simulink model "AA1111"  (R2018b)
settings: Solver=ode3  StartTime=0.0  StopTime=6000  FixedStep=T  RelTol=1e-3
PreLoadFcn:
  | Initial_LZ04
InitFcn:
  | Initial_LZ04
values from neighbouring files (symbols this model uses):
  Abg_GyroA = [0 0 1;0 1 0;-1 0 0]    [Initial_LZ04.m]
  Abg_GyroB = angle2dcm(-pi*3/4,0,-58/180*pi,'ZYX')    [Initial_LZ04.m]
  Abm_MmA = [0 -1 0;1 0 0;0 0 1]    [Initial_LZ04.m]
  Abm_MmB = [0 -1 0;1 0 0;0 0 1]    [Initial_LZ04.m]
  Att0 = 1*[80 0 0]'*pi/180    [Initial_LZ04.m]
  FixErr_StA = [15;15;15]*0*Kg_FixErr_St    [Initial_LZ04.m]
  FixErr_StB = ([15;15;15]*0+[10800;0;0])*Kg_FixErr_St    [Initial_LZ04.m]
  Fw_Mode = FW_Block(8,1)    [Initial.m]    (also in Initial_LZ04.m = 2)
  Fw_tao = 0.3    [Initial_LZ04.m]
  FwHmax = 4    [Initial_LZ04.m]
  FwTmax = FwTmax0    (= 0.05)    [Initial_LZ04.m]
  H0 = 0*[2;-2;-2;0]    [Initial_LZ04.m]
  Ib0_0 = [117.6 -1.39e-1 -1.14;-1.39e-1 101.9 -8.37e-2;-1.14 -8.37e-2 109.0]    [Initial_LZ04.m]
  jw = 0.0064    [Initial_LZ04.m]
  Matrix_I0 = [sin(50/180*pi)*cos(45/180*pi) -sin(50/180*pi)*cos(45/180*pi) -sin(50/180*pi)*cos(45/180*pi) sin(50/180*pi)*cos(45/180*pi);           sin(50/180*pi)*sin(45/180*pi) sin(50/180*pi)*sin(45/180*pi) -sin(50/180*pi)*sin(45/180*pi) -sin(50/180*pi)*sin(45/180*pi);           cos(50/180*pi) cos(50/180*pi) cos(50/180*pi) cos(50/180*pi)]    [Initial_LZ04.m]
  MtInfluence = 0    [Initial_LZ04.m]
  mu = 3.9860044e14    (= 398600440000000)    [Initial_LZ04.m]    (also in ZZ_User_Att.m)
  Ngc1 = [0.01;-0.02;-0.03]*Kg_Drift_Gyro*1+0*[0.001;-0.001;-0.001]    [Initial_LZ04.m]
  Ngc2 = [-0.02;0.01;-0.03]*Kg_Drift_Gyro    [Initial_LZ04.m]
  NgwxA = 0.005/60*sqrt(1/T_ctrl)*3*Kg_Noise_Gyro    [Initial_LZ04.m]
  NgwxB = 0.02/60*sqrt(1/T_ctrl)*3*Kg_Noise_Gyro    [Initial_LZ04.m]
  Noise_Mm = 7e-5*Kg_Noise_Mm    (= 7e-05)    [Initial_LZ04.m]
  Noise_StA = [3;3;30]*Kg_Noise_St    [Initial_LZ04.m]
  Noise_StB = [3;3;30]*Kg_Noise_St    [Initial_LZ04.m]
  OpenLoop_Att = 0    [Initial_LZ04.m]
  OpenLoop_Obt = 0    [Initial_LZ04.m]
  Qbs_StAFix = quatmultiply(angle2quat(pi,0,0,'XYZ'),angle2quat(-40/180*pi,20/180*pi,0,'XYZ'))    [Initial_LZ04.m]
  Qbs_StBFix = quatmultiply(angle2quat(pi,0,0,'XYZ'),angle2quat(40/180*pi,20/180*pi,0,'XYZ'))    [Initial_LZ04.m]
  Re = 6371.14e+3    (= 6371140)    [Initial.m]    (also in Initial_LZ04.m; ZZ_SystemApp.m)
  StartTime = [Year Month Day Hour Min Sec]'    [Initial_LZ04.m]
  T = T_PID - MainI.*[a_f/180*pi;0;0]    [Att_Ctrl.m]    (also in Initial_LZ04.m = 0.125; ZZ_Att.m = Tc(Axis))
  T_ctrl = 0.25    [Initial_LZ04.m]
  vx0 = sqrt(mu/a/(1-e^2))*(-sin(f)*sp(1)+(e+cos(f))*sq(1))    [Initial_LZ04.m]
  vy0 = sqrt(mu/a/(1-e^2))*(-sin(f)*sp(2)+(e+cos(f))*sq(2))    [Initial_LZ04.m]
  vz0 = sqrt(mu/a/(1-e^2))*(-sin(f)*sp(3)+(e+cos(f))*sq(3))    [Initial_LZ04.m]
  W_bi0 = 1*[0;-w0;0]+0*[2;-2;2]*pi/180    [Initial_LZ04.m]
  x0 = r0*(cos(omg+f)*cos(OMG)-sin(omg+f)*cos(i)*sin(OMG))    [Initial_LZ04.m]
  y0 = r0*(cos(omg+f)*sin(OMG)+sin(omg+f)*cos(i)*cos(OMG))    [Initial_LZ04.m]
  z0 = r0*sin(omg+f)*sin(i)    [Initial_LZ04.m]
undefined symbols (not defined in the file or in its folder): DiscIntNeverNeededParam, omegawXa
libraries: sharedutil x26, aerolibutil x15, simulink x12, sharedtransform x9, dspinverses x3, aerolibobsolete x1, vrlib x1
(part 2 of 3)

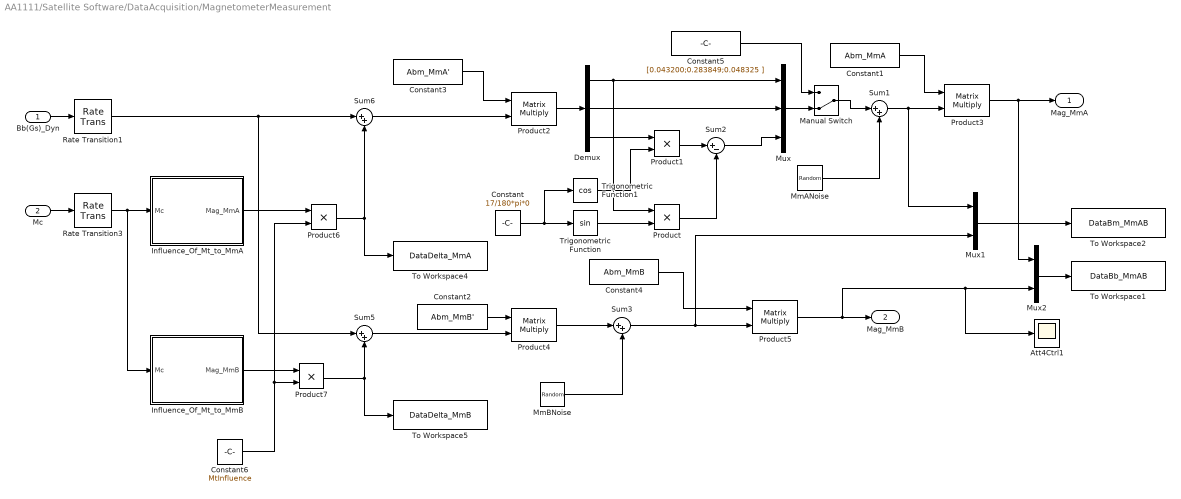
== system AA1111/Satellite Software/DataAcquisition/MagnetometerMeasurement ==
  Bb(Gs)_Dyn : Inport
  Mc : Inport  Port=2
  Att4Ctrl1 : Scope
  Constant : Constant  Value=17/180*pi*0
  Constant1 : Constant  Value=Abm_MmA
  Constant2 : Constant  Value=Abm_MmB'
  Constant3 : Constant  Value=Abm_MmA'
  Constant4 : Constant  Value=Abm_MmB
  Constant5 : Constant  Value=|
      | [0.043200;0.283849;0.048325
      | ]
  Constant6 : Constant  Value=MtInfluence
  Demux : Demux  Outputs=3
  Influence_Of_Mt_to_MmA : Subsystem
  Influence_Of_Mt_to_MmB : Subsystem
  Manual Switch : ManualSwitch  CurrentSetting=0
  MmANoise : RandomNumber  Mean=[0;0;0]  Variance=[(Noise_Mm/3)^2;(Noise_Mm/3)^2;(Noise_Mm/3)^2]  Seed=[100;111;112]  SampleTime=T_ctrl
  MmBNoise : RandomNumber  Mean=[0;0;0]  Variance=[(Noise_Mm/3)^2;(Noise_Mm/3)^2;(Noise_Mm/3)^2]  Seed=[10;11;12]  SampleTime=T_ctrl
  Mux : Mux  Inputs=3
  Mux1 : Mux  Inputs=2
  Mux2 : Mux  Inputs=2
  Product{,1,6..7} (4 alike) : Product  RndMeth=Zero
  Product{2..5} (4 alike) : Product  Multiplication=Matrix(*)  RndMeth=Zero
  Rate Transition1 : RateTransition  OutPortSampleTime=T_ctrl
  Rate Transition3 : RateTransition  OutPortSampleTime=T_ctrl
  Sum{1,3,5..6} (4 alike) : Sum  Inputs=|++
  Sum2 : Sum  Inputs=|+-
  To Workspace1 : ToWorkspace  VariableName=DataBb_MmAB  SampleTime=T_ctrl
  To Workspace2 : ToWorkspace  VariableName=DataBm_MmAB  SampleTime=T_ctrl
  To Workspace4 : ToWorkspace  VariableName=DataDelta_MmA  SampleTime=T_ctrl
  To Workspace5 : ToWorkspace  VariableName=DataDelta_MmB  SampleTime=T_ctrl
  Trigonometric Function : Trigonometry
  Trigonometric Function1 : Trigonometry  Operator=cos
  Mag_MmA : Outport
  Mag_MmB : Outport  Port=2
  wires:
  Demux/1 -> Mux/1, Product/1
  Demux/2 -> Mux/2
  Constant/1 -> Trigonometric Function/1, Trigonometric Function1/1
  Trigonometric Function/1 -> Product/2
  Demux/3 -> Product1/1
  Trigonometric Function1/1 -> Product1/2
  Product1/1 -> Sum2/1
  Product/1 -> Sum2/2
  Sum2/1 -> Mux/3
  Constant3/1 -> Product2/1
  Product2/1 -> Demux/1
  Bb(Gs)_Dyn/1 -> Rate Transition1/1
  Sum1/1 -> Product3/2, Mux1/1
  MmANoise/1 -> Sum1/2
  Constant2/1 -> Product4/1
  MmBNoise/1 -> Sum3/2
  Product4/1 -> Sum3/1
  Constant4/1 -> Product5/1
  Sum3/1 -> Product5/2, Mux1/2
  Product5/1 -> Mag_MmB/1, Mux2/2, Att4Ctrl1/1
  Constant1/1 -> Product3/1
  Product3/1 -> Mag_MmA/1, Mux2/1
  Mux1/1 -> To Workspace2/1
  Mux2/1 -> To Workspace1/1
  Mux/1 -> Manual Switch/2
  Manual Switch/1 -> Sum1/1
  Constant5/1 -> Manual Switch/1
  Sum6/1 -> Product2/2
  Influence_Of_Mt_to_MmA/1(Mag_MmA) -> Product6/1
  Influence_Of_Mt_to_MmB/1(Mag_MmB) -> Product7/1
  Sum5/1 -> Product4/2
  Mc/1 -> Rate Transition3/1
  Product7/1 -> Sum5/2, To Workspace5/1
  Product6/1 -> Sum6/2, To Workspace4/1
  Constant6/1 -> Product7/2, Product6/2
  Rate Transition1/1 -> Sum5/1, Sum6/1
  Rate Transition3/1 -> Influence_Of_Mt_to_MmA/1(Mc), Influence_Of_Mt_to_MmB/1(Mc)

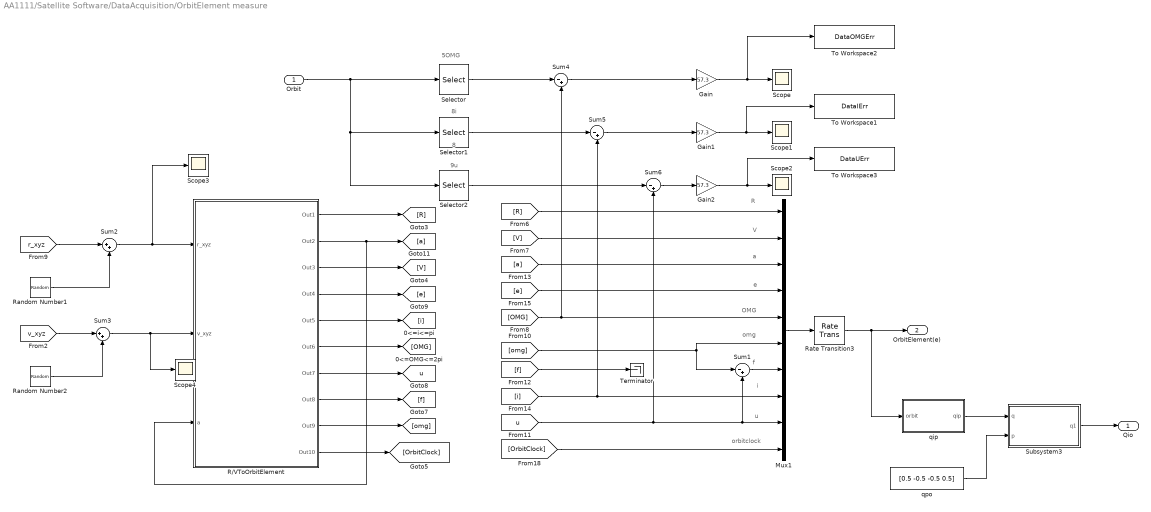
== system AA1111/Satellite Software/DataAcquisition/OrbitElement measure ==
  note: orbitclock
  note: u
  note: i
  note: f
  note: omg
  note: OMG
  note: e
  note: a
  note: V
  note: R
  note: 5OMG
  note: 9u
  note: 8
  note: 8i
  Orbit : Inport
  Gain : Gain  Gain=57.3
  Gain1 : Gain  Gain=57.3
  Gain2 : Gain  Gain=57.3
  Mux1 : Mux  Inputs=10
  R/VToOrbitElement : Subsystem
  Random Number1 : RandomNumber  Mean=[0;0;0]  Variance=([24;25;25]/3/2).^2  Seed=[13;14;15]  SampleTime=T_ctrl
  Random Number2 : RandomNumber  Mean=[0;0;0]  Variance=([0.15;0.15;0.15]/3/2).^2  Seed=[3;4;5]  SampleTime=T_ctrl
  Rate Transition3 : RateTransition  OutPortSampleTime=T_ctrl
  Scope{,1..4} (5 alike) : Scope
  Selector : Selector  InputPortWidth=10  IndexOptions=Index vector (dialog)  Indices=[5]  OutputSizes=1
  Selector1 : Selector  InputPortWidth=10  IndexOptions=Index vector (dialog)  Indices=[8]  OutputSizes=1
  Selector2 : Selector  InputPortWidth=10  IndexOptions=Index vector (dialog)  Indices=[9]  OutputSizes=1
  Subsystem3 : Subsystem
      mask Display: disp('quaternion\n multiply')
  Sum{1,4..6} (4 alike) : Sum  Inputs=|-+
  Sum2 : Sum  Inputs=|++
  Sum3 : Sum  Inputs=|++
  Terminator : Terminator
  To Workspace1 : ToWorkspace  VariableName=DataIErr  SampleTime=T_ctrl
  To Workspace2 : ToWorkspace  VariableName=DataOMGErr  SampleTime=T_ctrl
  To Workspace3 : ToWorkspace  VariableName=DataUErr  SampleTime=T_ctrl
  qip : Subsystem
  qpo : Constant  Value=[0.5 -0.5 -0.5 0.5]
  Qio : Outport
  OrbitElement(e) : Outport  Port=2
  tag scope: u=global
  wires:
  Subsystem3/1(q1) -> Qio/1
  qip/1(qip) -> Subsystem3/1(q)
  qpo/1 -> Subsystem3/2(p)
  Rate Transition3/1 -> OrbitElement(e)/1, qip/1(orbit)
  Mux1/1 -> Rate Transition3/1
  [u] -> Sum6/2, Mux1/9, Sum1/2
  [i] -> Sum5/2, Mux1/8
  [OMG] -> Mux1/5, Sum4/2
  [OrbitClock] -> Mux1/10
  [omg] -> Mux1/6, Sum1/1
  [e] -> Mux1/4
  [a] -> Mux1/3
  [V] -> Mux1/2
  [R] -> Mux1/1
  Sum1/1 -> Mux1/7
  [f] -> Terminator/1
  R/VToOrbitElement/1(Out1) -> [R]
  R/VToOrbitElement/2(Out2) -> R/VToOrbitElement/3(a), [a]
  R/VToOrbitElement/3(Out3) -> [V]
  R/VToOrbitElement/4(Out4) -> [e]
  R/VToOrbitElement/5(Out5) -> [i]
  R/VToOrbitElement/6(Out6) -> [OMG]
  R/VToOrbitElement/7(Out7) -> [u]
  R/VToOrbitElement/8(Out8) -> [f]
  R/VToOrbitElement/9(Out9) -> [omg]
  Orbit/1 -> Selector2/1, Selector1/1, Selector/1
  R/VToOrbitElement/10(Out10) -> [OrbitClock]
  [r_xyz] -> Sum2/1
  Random Number1/1 -> Sum2/2
  Sum2/1 -> Scope3/1, R/VToOrbitElement/1(r_xyz)
  [v_xyz] -> Sum3/1
  Sum3/1 -> Scope4/1, R/VToOrbitElement/2(v_xyz)
  Random Number2/1 -> Sum3/2
  Selector/1 -> Sum4/1
  Selector1/1 -> Sum5/1
  Selector2/1 -> Sum6/1
  Sum4/1 -> Gain/1
  Sum5/1 -> Gain1/1
  Sum6/1 -> Gain2/1
  Gain/1 -> To Workspace2/1, Scope/1
  Gain1/1 -> To Workspace1/1, Scope1/1
  Gain2/1 -> To Workspace3/1, Scope2/1

== system AA1111/Satellite Software/DataAcquisition/Star sensor measure ==
  note: qbs_StB
  note: qbs_StA
  note: qib
  note: qib
  Qib : Inport
  2 : Subsystem
  3 : Subsystem
  Constant : Constant  Value=Qbs_StAFix
  Constant1 : Constant  Value=Qbs_StBFix
  Q_StA_FixErr : Subsystem
  Q_StA_FixErr1 : Subsystem
  Quaternion Multiplication{,1..5} (6 alike) : aerolibutil/Quaternion Multiplication
  Quaternion Normalize : sharedutil/Quaternion Normalize  aMode=aMode
      settings: SourceProductName=Aerospace Blockset  SourceProductBaseCode=AE
  Quaternion Normalize1 : sharedutil/Quaternion Normalize  aMode=aMode
      settings: SourceProductName=Aerospace Blockset  SourceProductBaseCode=AE
  Rate Transition1 : RateTransition  OutPortSampleTime=T_ctrl
  Rate Transition2 : RateTransition  OutPortSampleTime=T_ctrl
  Qis_StA : Outport
  Qis_StB : Outport  Port=2
  wires:
  Quaternion Multiplication3/1 -> Rate Transition2/1
  Quaternion Multiplication2/1 -> Rate Transition1/1
  Quaternion Multiplication1/1 -> Quaternion Multiplication3/2
  Q_StA_FixErr1/1(Q_StB_FixErr) -> Quaternion Multiplication1/2
  Constant1/1 -> Quaternion Normalize1/1
  Q_StA_FixErr/1(Q_StA_FixErr) -> Quaternion Multiplication/2
  Constant/1 -> Quaternion Normalize/1
  3/1(q_StANoise) -> Quaternion Multiplication4/2
  2/1(q_StBNoise) -> Quaternion Multiplication5/2
  Quaternion Multiplication5/1 -> Qis_StB/1
  Quaternion Normalize/1 -> Quaternion Multiplication/1
  Quaternion Multiplication/1 -> Quaternion Multiplication2/2
  Quaternion Multiplication4/1 -> Qis_StA/1
  Rate Transition1/1 -> Quaternion Multiplication4/1
  Rate Transition2/1 -> Quaternion Multiplication5/1
  Quaternion Normalize1/1 -> Quaternion Multiplication1/1
  Qib/1 -> Quaternion Multiplication2/1, Quaternion Multiplication3/1

== system AA1111/Others/Attitude Kinematics Equations & Attitude Dynamics Equations/Kinetics/ECI TO ORBIT1 ==
  wbi(b) : Inport
  w00 : Inport  Port=2
  Abo : Inport  Port=3
  Constant : Constant  Value=0
  Gain : Gain  Gain=-1
  Matrix Multiply : Product  Multiplication=Matrix(*)
  Mux1 : Mux  Inputs=3
  Sum : Sum  Inputs=+|-
  wbo(b) : Outport
  wires:
  Mux1/1 -> Matrix Multiply/2
  w00/1 -> Gain/1
  Constant/1 -> Mux1/3, Mux1/1
  Gain/1 -> Mux1/2
  Abo/1 -> Matrix Multiply/1
  wbi(b)/1 -> Sum/1
  Sum/1 -> wbo(b)/1
  Matrix Multiply/1 -> Sum/2

== system AA1111/Others/Attitude Kinematics Equations & Attitude Dynamics Equations/Kinetics/ECI TO ORBIT2 ==
  wbi(b) : Inport
  w00 : Inport  Port=2
  Abo : Inport  Port=3
  Constant : Constant  Value=0
  Gain : Gain  Gain=-1
  Matrix Multiply : Product  Multiplication=Matrix(*)
  Mux1 : Mux  Inputs=3
  Sum : Sum  Inputs=+|-
  wbo(b) : Outport
  wires:
  Matrix Multiply/1 -> Sum/2
  Sum/1 -> wbo(b)/1
  wbi(b)/1 -> Sum/1
  Abo/1 -> Matrix Multiply/1
  Gain/1 -> Mux1/2
  Constant/1 -> Mux1/1, Mux1/3
  w00/1 -> Gain/1
  Mux1/1 -> Matrix Multiply/2

== system AA1111/Others/Attitude Kinematics Equations & Attitude Dynamics Equations/Kinetics/EulerIntegral ==
  w : Inport
  Abs : Abs
  Delay : Delay  DelayLength=1
  If : If  IfExpression=u1 > 0.0349
  If Action Subsystem : Subsystem  TreatAsAtomicUnit=on
  If Action Subsystem1 : Subsystem  TreatAsAtomicUnit=on
  Integrator : Integrator  ExternalReset=level  InitialCondition=Att0
  Merge : Merge
  Mux : Mux  Inputs=2
  OpenLoop : Constant  Value=OpenLoop_Att
  Selector : Selector  InputPortWidth=3  IndexOptions=Index vector (dialog)  Indices=[2]  OutputSizes=1
  Trigonometric Function : Trigonometry  Operator=cos
  W_Euler : Outport
  Agl_EulerInt : Outport  Port=2
  wires:
  w/1 -> Mux/1
  Trigonometric Function/1 -> Abs/1
  Abs/1 -> If/1
  If/1 -> If Action Subsystem/Action
  If/2 -> If Action Subsystem1/Action
  If Action Subsystem/1(Out1) -> Merge/1
  If Action Subsystem1/1(Out1) -> Merge/2
  Merge/1 -> W_Euler/1, Integrator/1, Delay/1
  Selector/1 -> Trigonometric Function/1
  Mux/1 -> If Action Subsystem/1(In1)
  Delay/1 -> If Action Subsystem1/1(In1)
  OpenLoop/1 -> Integrator/2
  Integrator/1 -> Agl_EulerInt/1, Selector/1, Mux/2

== system AA1111/Others/Attitude Kinematics Equations & Attitude Dynamics Equations/Kinetics/EulerIntegral1 ==
  w : Inport
  Agl0_Inertial : Inport  Port=2
  Abs : Abs
  Delay : Delay  DelayLength=1
  If : If  IfExpression=u1 > 0.0349
  If Action Subsystem : Subsystem  TreatAsAtomicUnit=on
  If Action Subsystem1 : Subsystem  TreatAsAtomicUnit=on
  Integrator : Integrator  ExternalReset=level  InitialConditionSource=external
  Merge : Merge
  Mux : Mux  Inputs=2
  OpenLoop : Constant  Value=OpenLoop_Att
  Selector : Selector  InputPortWidth=3  IndexOptions=Index vector (dialog)  Indices=[2]  OutputSizes=1
  Trigonometric Function : Trigonometry  Operator=cos
  Agl_EulerInt : Outport
  wires:
  Integrator/1 -> Mux/2, Selector/1, Agl_EulerInt/1
  OpenLoop/1 -> Integrator/2
  Delay/1 -> If Action Subsystem1/1(In1)
  Mux/1 -> If Action Subsystem/1(In1)
  Selector/1 -> Trigonometric Function/1
  Merge/1 -> Delay/1, Integrator/1
  If Action Subsystem1/1(Out1) -> Merge/2
  If Action Subsystem/1(Out1) -> Merge/1
  If/2 -> If Action Subsystem1/Action
  If/1 -> If Action Subsystem/Action
  Abs/1 -> If/1
  Trigonometric Function/1 -> Abs/1
  w/1 -> Mux/1
  Agl0_Inertial/1 -> Integrator/3

== system AA1111/Others/Attitude Kinematics Equations & Attitude Dynamics Equations/Kinetics/Qob 2 Qib ==
  note: qio
  note: qib
  note: qob
  note: µØÐÄ¹ìµÀÏµ¡úo
  note: qib=qip*qpo*qob
  note: iÎªµØÐÄ¹ßÐÔÏµ
      | pÎªµØÐÄ¹ìµÀÏµ
      | oÎªÎÀÐÇ¹ìµÀÏµ
      | bÎªÎÀÐÇ±¾ÌåÏµ
  Qob : Inport
  OrbitElement : Inport  Port=2
  Display1 : Display
  Quaternion Multiplication : aerolibutil/Quaternion Multiplication
  Quaternion Multiplication1 : aerolibutil/Quaternion Multiplication
  qip : Subsystem
  qpo : Constant  Value=[0.5 -0.5 -0.5 0.5]
  qib : Outport
  wires:
  Quaternion Multiplication1/1 -> qib/1
  qip/1(qip) -> Quaternion Multiplication/1
  qpo/1 -> Quaternion Multiplication/2
  Quaternion Multiplication/1 -> Quaternion Multiplication1/1, Display1/1
  Qob/1 -> Quaternion Multiplication1/2
  OrbitElement/1 -> qip/1(orbit)

== system AA1111/Others/Attitude Kinematics Equations & Attitude Dynamics Equations/Kinetics/Qob 2 Qib1 ==
  note: iÎªµØÐÄ¹ßÐÔÏµ
      | pÎªµØÐÄ¹ìµÀÏµ
      | oÎªÎÀÐÇ¹ìµÀÏµ
      | bÎªÎÀÐÇ±¾ÌåÏµ
  note: qib=qip*qpo*qob
  note: µØÐÄ¹ìµÀÏµ¡úo
  note: qob
  note: qib
  note: qio
  Qob : Inport
  OrbitElement : Inport  Port=2
  Quaternion Multiplication : aerolibutil/Quaternion Multiplication
  Quaternion Multiplication1 : aerolibutil/Quaternion Multiplication
  qip : Subsystem
  qpo : Constant  Value=[0.5 -0.5 -0.5 0.5]
  qib : Outport
  wires:
  OrbitElement/1 -> qip/1(orbit)
  Qob/1 -> Quaternion Multiplication1/2
  Quaternion Multiplication/1 -> Quaternion Multiplication1/1
  qpo/1 -> Quaternion Multiplication/2
  qip/1(qip) -> Quaternion Multiplication/1
  Quaternion Multiplication1/1 -> qib/1

== system AA1111/Others/Attitude Kinematics Equations & Attitude Dynamics Equations/Kinetics/Quaternion Kinematics ==
  wbo(b) : Inport
  Agl0 : Constant  Value=Att0
  Discrete-Time Integrator : DiscreteIntegrator  ExternalReset=level  InitialConditionSource=external  InitialCondition=[1;0;0;0]  SampleTime=T  ICPrevOutput=DiscIntNeverNeededParam  ICPrevScaledInput=DiscIntNeverNeededParam
  Mux : Mux  Inputs=2
  Mux1 : Mux
  OpenLoop : Constant  Value=OpenLoop_Att
  Quaternion Normalize : sharedutil/Quaternion Normalize  aMode=aMode
      settings: SourceProductName=Aerospace Blockset  SourceProductBaseCode=AE
  Rotation Angles to Quaternions : sharedtransform/Rotation Angles to Quaternions  rotationOrder=ZYX  aMode=aMode
      settings: SourceProductName=Aerospace Blockset  SourceProductBaseCode=AE
  Selector : Selector  InputPortWidth=3  IndexOptions=Index vector (dialog)  Indices=[3 2 1]  OutputSizes=1
  dq0/dt : Fcn  Expr=0.5*(-u(1)*u(5)-u(2)*u(6)-u(3)*u(7))
  dq1/dt : Fcn  Expr=0.5*(u(1)*u(4)+u(3)*u(6)-u(2)*u(7))
  dq2/dt : Fcn  Expr=0.5*(u(2)*u(4)-u(3)*u(5)+u(1)*u(7))
  dq3/dt : Fcn  Expr=0.5*(u(3)*u(4)+u(2)*u(5)-u(1)*u(6))
  qob : Outport
  wires:
  wbo(b)/1 -> Mux/1
  Mux1/1 -> Discrete-Time Integrator/1
  Quaternion Normalize/1 -> Mux/2, qob/1
  dq0/dt/1 -> Mux1/1
  dq1/dt/1 -> Mux1/2
  dq2/dt/1 -> Mux1/3
  dq3/dt/1 -> Mux1/4
  Mux/1 -> dq2/dt/1, dq3/dt/1, dq1/dt/1, dq0/dt/1
  Agl0/1 -> Selector/1
  Discrete-Time Integrator/1 -> Quaternion Normalize/1
  Rotation Angles to Quaternions/1 -> Discrete-Time Integrator/3
  Selector/1 -> Rotation Angles to Quaternions/1
  OpenLoop/1 -> Discrete-Time Integrator/2

== system AA1111/Others/Attitude Kinematics Equations & Attitude Dynamics Equations/Kinetics/between-2pi//3and4pi//3 ==
  in : Inport
  Compare To Constant : simulink/Logic and Bit Operations/Compare To Constant  relop=<  const=-2  OutDataTypeStr=uint8
  Compare To Constant1 : simulink/Logic and Bit Operations/Compare To Constant  relop=<  const=-2  OutDataTypeStr=uint8
  Compare To Constant2 : simulink/Logic and Bit Operations/Compare To Constant  relop=<  const=-2  OutDataTypeStr=uint8
  Constant : Constant  Value=2*pi
  Constant1 : Constant  Value=2*pi
  Constant2 : Constant  Value=2*pi
  Demux : Demux  Outputs=3
  Mux1 : Mux  Inputs=3
  Product : Product  RndMeth=Zero
  Product1 : Product  RndMeth=Zero
  Product2 : Product  RndMeth=Zero
  Sum : Sum  Inputs=|++
  Sum1 : Sum  Inputs=++|
  Sum2 : Sum
  out : Outport
  wires:
  Mux1/1 -> out/1
  Compare To Constant2/1 -> Product2/2
  Constant2/1 -> Product2/1
  Sum2/1 -> Mux1/2
  Product2/1 -> Sum2/2
  Demux/2 -> Compare To Constant2/1, Sum2/1
  Sum/1 -> Mux1/3
  Product1/1 -> Sum/2
  Constant1/1 -> Product1/2
  Compare To Constant1/1 -> Product1/1
  Sum1/1 -> Mux1/1
  Product/1 -> Sum1/1
  Compare To Constant/1 -> Product/2
  Constant/1 -> Product/1
  Demux/1 -> Compare To Constant/1, Sum1/2
  Demux/3 -> Compare To Constant1/1, Sum/1
  in/1 -> Demux/1

== system AA1111/Others/Disturbing torque/Compute JD/Subsystem1 ==
  note: Y
  note: M
  note: D
  note: 3
  note: 1
  note: 2
  In : Inport
  Add : Sum  Inputs=+++--
  Constant1 : Constant  Value=0.5
  Fcn1 : Fcn  Expr=(u(1)-14)/12
  Fcn2 : Fcn  Expr=1461*(u(1)+4800+u(2))/4
  Fcn3 : Fcn  Expr=367*(u(1)-2-u(2)*12)/12
  Fcn4 : Fcn  Expr=(u(1)+4900+u(2))/100
  Fcn5 : Fcn  Expr=3*u(1)/4
  Fcn6 : Fcn  Expr=u(1)-32075
  Mux : Mux  Inputs=2
  Mux1 : Mux  Inputs=2
  Rounding Function{1..5} (5 alike) : Rounding  Operator=fix
  Selector : Selector  InputPortWidth=3  IndexOptions=Index vector (dialog)  Indices=[1]  OutputSizes=1
  Selector1 : Selector  InputPortWidth=3  IndexOptions=Index vector (dialog)  Indices=[2]  OutputSizes=1
  Selector2 : Selector  InputPortWidth=3  IndexOptions=Index vector (dialog)  Indices=[3]  OutputSizes=1
  Out : Outport
  wires:
  Add/1 -> Out/1
  In/1 -> Selector/1, Selector1/1, Selector2/1
  Selector1/1 -> Fcn1/1, Mux1/1
  Fcn1/1 -> Rounding Function1/1
  Rounding Function1/1 -> Mux/2, Mux1/2
  Selector/1 -> Mux/1
  Mux/1 -> Fcn2/1, Fcn4/1
  Fcn2/1 -> Rounding Function2/1
  Mux1/1 -> Fcn3/1
  Fcn3/1 -> Rounding Function3/1
  Fcn4/1 -> Rounding Function4/1
  Rounding Function4/1 -> Fcn5/1
  Fcn5/1 -> Rounding Function5/1
  Selector2/1 -> Fcn6/1
  Fcn6/1 -> Add/1
  Rounding Function2/1 -> Add/2
  Rounding Function3/1 -> Add/3
  Rounding Function5/1 -> Add/4
  Constant1/1 -> Add/5

== system AA1111/Others/Disturbing torque/Compute geomagnetism1/Subsystem ==
  note: ³àÎ³
  note: u
  note: i
  Orbit : Inport
  JDC : Inport  Port=2
  Constant : Constant  Value=pi/2
  Fcn1 : Fcn  Expr=u(9)
  Fcn13 : Fcn  Expr=(18.6973746+879000.0513367*u(1)+(0.093104*u(1)^2-6.2e-6*u(1)^3)/3600.0*0)*360.0/24.0*pi/180
  Fcn5 : Fcn  Expr=asin(sin(u[1])*sin(u[2]))
  Fcn8 : Fcn  Expr=u(8)
  Gain2 : Gain
  Gain3 : Gain  Gain=180/pi
  I_Long : Terminator
  Mux4 : Mux  Inputs=2
  Subsystem1 : Subsystem
  Sum : Sum  Inputs=|-+
  Lat. : Outport
  G_Long. : Outport  Port=2
  YuWei : Outport  Port=3
  wires:
  Gain2/1 -> G_Long./1
  Sum/1 -> YuWei/1
  Constant/1 -> Sum/2
  Gain3/1 -> I_Long/1
  Subsystem1/2(I_Long) -> Gain3/1
  JDC/1 -> Fcn13/1
  Fcn13/1 -> Subsystem1/1(GAST)
  Fcn1/1 -> Mux4/1
  Subsystem1/1(G_Long.) -> Gain2/1
  Fcn5/1 -> Lat./1, Sum/1, Subsystem1/3(Lat.)
  Orbit/1 -> Fcn8/1, Fcn1/1, Subsystem1/2(OrbitElement)
  Mux4/1 -> Fcn5/1
  Fcn8/1 -> Mux4/2

== system AA1111/Others/Disturbing torque/Compute geomagnetism1/Transfer Matrix ==
  note: Aop
  note: µØ´ÅÏµ2¹ìµÀÏµ£¿£¿£¿
  note: u
  note: i
  Abo : Inport
  Orbit : Inport  Port=2
  DiXinLatitude : Inport  Port=3
  Aop1 : Subsystem
  Constant : Constant  Value=pi/2
  Divide : Product  Inputs=*/
  Fcn1 : Fcn  Expr=u(9)
  Fcn8 : Fcn  Expr=u(8)
  "From Northt_East_down 2 body  " : Product  Multiplication=Matrix(*)  SaturateOnIntegerOverflow=on  OutDataTypeStr=Inherit: Same as first input
  Gain : Gain  Gain=-1
  If : If
  If Action Subsystem : Subsystem  TreatAsAtomicUnit=on
  If Action Subsystem1 : Subsystem  TreatAsAtomicUnit=on
  Manual Switch : ManualSwitch  CurrentSetting=0
  Merge : Merge
  Mux : Mux  Inputs=2
  O-NEG : Subsystem
  Sum : Sum  Inputs=|-+
  Trigonometric Function : Trigonometry
  Trigonometric Function1 : Trigonometry  Operator=cos
  Trigonometric Function2 : Trigonometry  Operator=asin
  Trigonometric Function3 : Trigonometry  Operator=cos
  Aop : Outport
  Abp : Outport  Port=2
  wires:
  Aop1/1(Out1) -> Manual Switch/2
  Manual Switch/1 -> "From Northt_East_down 2 body  "/2, Aop/1
  Merge/1 -> Aop1/1(In1)
  If Action Subsystem1/1(Out1) -> Merge/2
  If Action Subsystem/1(Out1) -> Merge/1
  If/2 -> If Action Subsystem1/Action
  Trigonometric Function2/1 -> If Action Subsystem1/1(In1), If Action Subsystem/1(In1)
  If/1 -> If Action Subsystem/Action
  Trigonometric Function3/1 -> If/1
  Divide/1 -> Trigonometric Function2/1
  Trigonometric Function/1 -> Divide/2
  Gain/1 -> Divide/1
  Trigonometric Function1/1 -> Gain/1
  Sum/1 -> Trigonometric Function/1
  Constant/1 -> Sum/2
  DiXinLatitude/1 -> Sum/1
  "From Northt_East_down 2 body  "/1 -> Abp/1
  O-NEG/1(Out1) -> Manual Switch/1
  Mux/1 -> O-NEG/1(In1)
  Fcn1/1 -> Trigonometric Function3/1, Mux/2
  Fcn8/1 -> Trigonometric Function1/1, Mux/1
  Abo/1 -> "From Northt_East_down 2 body  "/1
  Orbit/1 -> Fcn1/1, Fcn8/1

== system AA1111/Others/Oribit motion model/Compute osculating elements/  ==
  note: 0<=OMG<=2pi
  Hi : Inport
  Fcn1 : Fcn  Expr=u(1)
  Fcn2 : Fcn  Expr=u(2)
  If : If  IfExpression=u1 < 0
  If Action Subsystem : Subsystem  TreatAsAtomicUnit=on
  If Action Subsystem1 : Subsystem  TreatAsAtomicUnit=on
  Merge : Merge
  Mux3 : Mux  Inputs=2
  tg(OMG)=Hxi/(-Hyi) : Fcn  Expr=atan2(u[1],-u[2])
  OMG : Outport
  wires:
  Fcn1/1 -> Mux3/1
  Fcn2/1 -> Mux3/2
  Mux3/1 -> tg(OMG)=Hxi/(-Hyi)/1
  tg(OMG)=Hxi/(-Hyi)/1 -> If/1, If Action Subsystem/1(In1), If Action Subsystem1/1(In1)
  If/1 -> If Action Subsystem/Action
  If/2 -> If Action Subsystem1/Action
  If Action Subsystem/1(Out1) -> Merge/1
  If Action Subsystem1/1(Out1) -> Merge/2
  Merge/1 -> OMG/1
  Hi/1 -> Fcn1/1, Fcn2/1

== system AA1111/Others/Oribit motion model/Compute osculating elements/      ==
  H_xyz : Inport
  R_xyz : Inport  Port=2
  3x3 Cross Product : sharedutil/3x3 Cross Product  aMode=aMode
      settings: SourceProductBaseCode=AE
  Dot Product4 : DotProduct  InputSameDT=on  OutDataTypeStr=Inherit: Inherit via internal rule
  Fcn1 : Fcn  Expr=acos(u[2]/(u[1]*u[3]))
  Fcn3 : Fcn  Expr=sqrt(u[1]^2+u[2]^2+u[3]^2)
  Fcn4 : Fcn  Expr=u[3]
  Fcn5 : Fcn  Expr=sqrt(u[1]^2+u[2]^2+u[3]^2)
  If Action Subsystem2 : Subsystem  TreatAsAtomicUnit=on
  If Action Subsystem3 : Subsystem  TreatAsAtomicUnit=on
  If1 : If
  Merge1 : Merge
  Mux1 : Mux  Inputs=3
  uz : Constant  Value=[0;0;1]  VectorParams1D=off
  u : Outport
  wires:
  uz/1 -> 3x3 Cross Product/1
  H_xyz/1 -> 3x3 Cross Product/2
  3x3 Cross Product/1 -> Dot Product4/1, Fcn5/1
  R_xyz/1 -> Fcn3/1, Dot Product4/2, Fcn4/1
  Fcn3/1 -> Mux1/3
  Dot Product4/1 -> Mux1/2
  Mux1/1 -> Fcn1/1
  Fcn4/1 -> If1/1
  If1/1 -> If Action Subsystem2/Action
  Fcn1/1 -> If Action Subsystem2/1(In1), If Action Subsystem3/1(In1)
  If Action Subsystem2/1(Out1) -> Merge1/1
  If Action Subsystem3/1(Out1) -> Merge1/2
  Merge1/1 -> u/1
  Fcn5/1 -> Mux1/1
  If1/2 -> If Action Subsystem3/Action

== system AA1111/Others/Oribit motion model/Compute osculating elements/     1 ==
  note: Orbit Period T
  u : Inport
  a : Inport  Port=2
  Fcn : Fcn  Expr=2*pi*sqrt(u(1)^3/mu)
  If Action Subsystem1 : Subsystem  TreatAsAtomicUnit=on
  If Action Subsystem2 : Subsystem  TreatAsAtomicUnit=on
  If1 : If  IfExpression=u1 <pi
  Merge1 : Merge
  OrbitClock : Outport
  wires:
  If1/2 -> If Action Subsystem1/Action
  Merge1/1 -> OrbitClock/1
  If Action Subsystem1/1(Out1) -> Merge1/2
  If Action Subsystem2/1(Out1) -> Merge1/1
  If1/1 -> If Action Subsystem2/Action
  u/1 -> If Action Subsystem2/1(u), If1/1, If Action Subsystem1/1(u)
  a/1 -> Fcn/1
  Fcn/1 -> If Action Subsystem2/2(T), If Action Subsystem1/2(T)

== system AA1111/Others/Oribit motion model/Compute osculating elements/   1 ==
  note: 0<=omg<=2pi
  note: Éý½»µãÊ¸Á¿Óë½üµØµãÊ¸Á¿µÄ¼Ð½Ç
  note: ¹ìµÀ½ÚÏßÊ¸Á¿N
  H_xyz : Inport
  V_xyz : Inport  Port=2
  R_xyz : Inport  Port=3
  3x3 Cross Product : sharedutil/3x3 Cross Product  aMode=aMode
      settings: SourceProductBaseCode=AE
  3x3 Cross Product1 : sharedutil/3x3 Cross Product  aMode=aMode
      settings: SourceProductBaseCode=AE
  Divide : Product  Inputs=*/
  Dot Product3 : DotProduct  InputSameDT=on  OutDataTypeStr=Inherit: Inherit via internal rule
  Fcn : Fcn  Expr=acos(u[2]/(u[1]*u[3]))
  Fcn2 : Fcn  Expr=u[3]
  Fcn3 : Fcn  Expr=sqrt(u[1]^2+u[2]^2+u[3]^2)
  Fcn5 : Fcn  Expr=sqrt(u[1]^2+u[2]^2+u[3]^2)
  Fcn6 : Fcn  Expr=sqrt(u[1]^2+u[2]^2+u[3]^2)
  Gain1 : Gain  Gain=180/pi
  Gain3 : Gain  Gain=mu  SaturateOnIntegerOverflow=on  OutDataTypeStr=Inherit: Same as input  ParamDataTypeStr=Inherit: Same as input
  If : If  IfExpression=u1 >= 0
  If Action Subsystem : Subsystem  TreatAsAtomicUnit=on
  If Action Subsystem1 : Subsystem  TreatAsAtomicUnit=on
  Merge : Merge
  Mux : Mux  Inputs=3
  Sum : Sum  Inputs=|--  SaturateOnIntegerOverflow=on
  uz : Constant  Value=[0;0;1]  VectorParams1D=off
  w{,1..4} (5 alike) : Scope
  omg : Outport
  wires:
  H_xyz/1 -> 3x3 Cross Product/2, 3x3 Cross Product1/1
  If Action Subsystem1/1(Out1) -> Merge/2
  If Action Subsystem/1(Out1) -> Merge/1
  Fcn/1 -> If Action Subsystem1/1(In1), If Action Subsystem/1(In1), Gain1/1
  Fcn2/1 -> If/1, w1/1
  Mux/1 -> Fcn/1
  Fcn6/1 -> Mux/3, w4/1
  Sum/1 -> Fcn2/1, Dot Product3/2, Fcn6/1
  Divide/1 -> Sum/2, w2/1
  Fcn3/1 -> Divide/2
  3x3 Cross Product/1 -> Fcn5/1, Dot Product3/1
  uz/1 -> 3x3 Cross Product/1
  3x3 Cross Product1/1 -> Sum/1, w3/1
  R_xyz/1 -> Fcn3/1, Gain3/1
  Dot Product3/1 -> Mux/2
  V_xyz/1 -> 3x3 Cross Product1/2
  Merge/1 -> omg/1
  If/1 -> If Action Subsystem/Action
  If/2 -> If Action Subsystem1/Action
  Gain1/1 -> w/1
  Gain3/1 -> Divide/1
  Fcn5/1 -> Mux/1

== system AA1111/Satellite Software/DataAcquisition/GyroMeasurment/TurntableModel ==
  wbi : Inport
  Demux : Demux  Outputs=3
  Demux1 : Demux  Outputs=3
  GyroOnTurntable : Subsystem
  Mux{,1..3} (4 alike) : Mux  Inputs=2
  To Workspace1 : ToWorkspace  VariableName=DataGyro_TurnTable  SampleTime=T_ctrl
  To Workspace2 : ToWorkspace  VariableName=DataAtt_TurnTable  SampleTime=T_ctrl
  Turntable Model : Subsystem
  TurntableRotateSpeedCal : Subsystem
  deg2rad : Gain  Gain=pi/180
  dphi : Scope
  phi : Scope
  rad2deg : Gain  Gain=180/pi
  w : Scope  NumInputPorts=3
  wbi_out : Outport
  wires:
  TurntableRotateSpeedCal/1(dfai(¡ã/s)) -> Turntable Model/1(W(¡ã/s)), GyroOnTurntable/1(dfai(¡ã/s)), dphi/1, Mux3/2
  Turntable Model/1(Angle(¡ã)) -> phi/1, TurntableRotateSpeedCal/2(angle(¡ã)), GyroOnTurntable/2(angle(¡ã)), Mux3/1
  wbi/1 -> rad2deg/1
  rad2deg/1 -> TurntableRotateSpeedCal/1(wbi(¡ã/s)), Demux1/1
  GyroOnTurntable/1(wbi(¡ã/s)) -> Demux/1, To Workspace1/1, deg2rad/1
  Demux/1 -> Mux/1
  Demux1/1 -> Mux/2
  Demux/2 -> Mux1/1
  Demux1/2 -> Mux1/2
  Demux/3 -> Mux2/1
  Demux1/3 -> Mux2/2
  Mux/1 -> w/1
  Mux1/1 -> w/2
  Mux2/1 -> w/3
  Mux3/1 -> To Workspace2/1
  deg2rad/1 -> wbi_out/1

== system AA1111/Satellite Software/DataAcquisition/MagnetometerMeasurement/Influence_Of_Mt_to_MmA ==
  note: 100mAµÄ´ÅÁ¦¾ØÆ÷x
      | ÔÚ´ÅÇ¿¼ÆA´¦²úÉúµÄ´Å³¡
      | ÔÚ±¾ÌåÏµÏÂµÄ±íÊ¾
  Mc : Inport
  Constant1 : Constant  Value=[-0.0160;-0.0090;-0.0110]
  Constant2 : Constant  Value=[0.0045;-0.0270;-0.0605]
  Constant4 : Constant  Value=[-0.0185;0.0155;-0.0590]
  Demux2 : Demux  Outputs=3
  Gain3 : Gain  Gain=1/25
  Product1 : Product  RndMeth=Zero
  Product2 : Product  RndMeth=Zero
  Product3 : Product  RndMeth=Zero
  Sum1 : Sum  Inputs=+++
  Mag_MmA : Outport
  wires:
  Sum1/1 -> Mag_MmA/1
  Constant4/1 -> Product1/1
  Constant2/1 -> Product2/1
  Constant1/1 -> Product3/1
  Product1/1 -> Sum1/1
  Product2/1 -> Sum1/2
  Demux2/2 -> Product2/2
  Demux2/3 -> Product3/2
  Demux2/1 -> Product1/2
  Gain3/1 -> Demux2/1
  Product3/1 -> Sum1/3
  Mc/1 -> Gain3/1

== system AA1111/Satellite Software/DataAcquisition/MagnetometerMeasurement/Influence_Of_Mt_to_MmB ==
  note: 100mAµÄ´ÅÁ¦¾ØÆ÷x
      | ÔÚ´ÅÇ¿¼ÆB´¦²úÉúµÄ´Å³¡
      | ÔÚ±¾ÌåÏµÏÂµÄ±íÊ¾
  Mc : Inport
  Constant1 : Constant  Value=[-0.0270;0.0055;-0.0120]
  Constant2 : Constant  Value=[-0.0030;-0.0165;0.0660]
  Constant4 : Constant  Value=[-0.0155;-0.0195;-0.0260]
  Demux1 : Demux  Outputs=3
  Gain : Gain  Gain=1/25
  Product : Product  RndMeth=Zero
  Product10 : Product  RndMeth=Zero
  Product11 : Product  RndMeth=Zero
  Sum6 : Sum  Inputs=+++
  Mag_MmB : Outport
  wires:
  Sum6/1 -> Mag_MmB/1
  Constant4/1 -> Product/1
  Constant2/1 -> Product10/1
  Constant1/1 -> Product11/1
  Product/1 -> Sum6/1
  Product10/1 -> Sum6/2
  Demux1/2 -> Product10/2
  Demux1/3 -> Product11/2
  Mc/1 -> Gain/1
  Demux1/1 -> Product/2
  Gain/1 -> Demux1/1
  Product11/1 -> Sum6/3

== system AA1111/Satellite Software/DataAcquisition/OrbitElement measure/R//VToOrbitElement ==
  note: µØÐÄ¹ìµÀÏµ¡úo
  note: acos's range: [0 pi]
  note: Hi
  r_xyz : Inport
  v_xyz : Inport  Port=2
  a : Inport  Port=3
  " " : Subsystem
  "     " : Subsystem
  "     1" : Subsystem
  "   1" : Subsystem
  3x3 Cross Product : sharedutil/3x3 Cross Product  aMode=aMode
      settings: SourceProductBaseCode=AE
  Fcn : Fcn  Expr=-0.5*mu/(u[2]^2/2-mu/u[1])
  Fcn1 : Fcn  Expr=sqrt(1-u[2]^2/mu/u[1])
  Fcn2 : Fcn  Expr=acos(u[2]/u[1])
  Fcn3 : Fcn  Expr=sqrt(u[1]^2+u[2]^2+u[3]^2)
  Fcn4 : Fcn  Expr=sqrt(u[1]^2+u[2]^2+u[3]^2)
  Hzi : Fcn  Expr=u[3]
  Mux : Mux  Inputs=2
  Mux2 : Mux  Inputs=2
  Mux3 : Mux  Inputs=2
  Sum : Sum  Inputs=+-
  |H| : Fcn  Expr=sqrt(u[1]^2+u[2]^2+u[3]^2)
  Out1 : Outport
  Out2 : Outport  Port=2
  Out3 : Outport  Port=3
  Out4 : Outport  Port=4
  Out5 : Outport  Port=5
  Out6 : Outport  Port=6
  Out7 : Outport  Port=7
  Out8 : Outport  Port=8
  Out9 : Outport  Port=9
  Out10 : Outport  Port=10
  wires:
  Mux3/1 -> Fcn2/1
  "     "/1(u) -> "     1"/1(u), Out7/1, Sum/1
  Fcn3/1 -> Out1/1, Mux/1
  Hzi/1 -> Mux3/2
  "   1"/1(omg) -> Out9/1, Sum/2
  3x3 Cross Product/1 -> |H|/1, " "/1(Hi), "     "/1(H_xyz), "   1"/1(H_xyz), Hzi/1
  |H|/1 -> Mux2/2, Mux3/1
  Fcn4/1 -> Out3/1, Mux/2
  Mux2/1 -> Fcn1/1
  a/1 -> Mux2/1, "     1"/2(a)
  Fcn2/1 -> Out5/1
  r_xyz/1 -> Fcn3/1, "     "/2(R_xyz), "   1"/3(R_xyz), 3x3 Cross Product/1
  "     1"/1(OrbitClock) -> Out10/1
  Mux/1 -> Fcn/1
  " "/1(OMG) -> Out6/1
  Sum/1 -> Out8/1
  Fcn/1 -> Out2/1
  v_xyz/1 -> "   1"/2(V_xyz), 3x3 Cross Product/2, Fcn4/1
  Fcn1/1 -> Out4/1

== system AA1111/Satellite Software/DataAcquisition/OrbitElement measure/Subsystem3 ==
  note: q1=q*p
  q : Inport
  p : Inport  Port=2
  0 : Fcn  Expr=u(1)*u(5)-u(2)*u(6)-u(3)*u(7)-u(4)*u(8)
  1 : Fcn  Expr=u(1)*u(6)+u(2)*u(5)+u(3)*u(8)-u(4)*u(7)
  2 : Fcn  Expr=u(1)*u(7)-u(2)*u(8)+u(3)*u(5)+u(4)*u(6)
  3 : Fcn  Expr=u(1)*u(8)+u(2)*u(7)-u(3)*u(6)+u(4)*u(5)
  Demux1 : Demux
  Demux2 : Demux
  Mux : Mux
  Mux1 : Mux  Inputs=8
  Quaternion Normalize : sharedutil/Quaternion Normalize  aMode=aMode
      settings: SourceProductName=Aerospace Blockset  SourceProductBaseCode=AE
  q1 : Outport
  wires:
  Quaternion Normalize/1 -> q1/1
  q/1 -> Demux2/1
  Mux/1 -> Quaternion Normalize/1
  p/1 -> Demux1/1
  0/1 -> Mux/1
  1/1 -> Mux/2
  2/1 -> Mux/3
  3/1 -> Mux/4
  Demux2/1 -> Mux1/1
  Demux2/2 -> Mux1/2
  Demux2/3 -> Mux1/3
  Demux2/4 -> Mux1/4
  Demux1/1 -> Mux1/5
  Demux1/2 -> Mux1/6
  Demux1/3 -> Mux1/7
  Demux1/4 -> Mux1/8
  Mux1/1 -> 0/1, 1/1, 2/1, 3/1

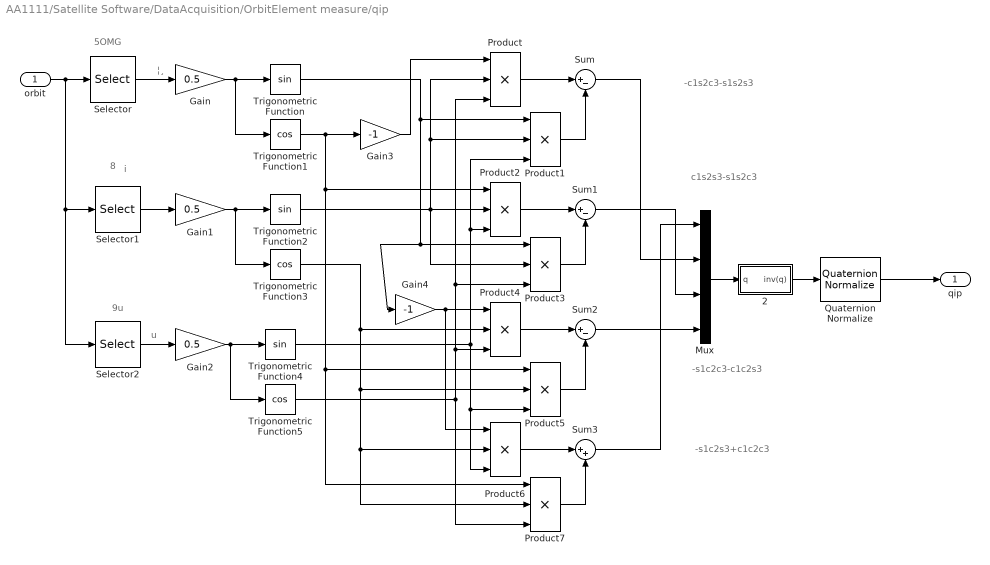
== system AA1111/Satellite Software/DataAcquisition/OrbitElement measure/qip ==
  note: -s1c2s3+c1c2c3
  note: -s1c2c3-c1c2s3
  note: c1s2s3-s1s2c3
  note: -c1s2c3-s1s2s3
  note: 9u
  note: 8
  note: 5OMG
  note: u
  note: i
  note: ¦¸
  orbit : Inport
  2 : Subsystem
      mask Display: disp(' ')
  Gain : Gain  Gain=0.5
  Gain1 : Gain  Gain=0.5
  Gain2 : Gain  Gain=0.5
  Gain3 : Gain  Gain=-1
  Gain4 : Gain  Gain=-1
  Mux : Mux
  Product{,1..7} (8 alike) : Product  Inputs=3  RndMeth=Zero
  Quaternion Normalize : sharedutil/Quaternion Normalize  aMode=aMode
      settings: SourceProductName=Aerospace Blockset  SourceProductBaseCode=AE
  Selector : Selector  InputPortWidth=10  IndexOptions=Index vector (dialog)  Indices=[5]  OutputSizes=1
  Selector1 : Selector  InputPortWidth=10  IndexOptions=Index vector (dialog)  Indices=[8]  OutputSizes=1
  Selector2 : Selector  InputPortWidth=10  IndexOptions=Index vector (dialog)  Indices=[9]  OutputSizes=1
  Sum : Sum  Inputs=|+-
  Sum1 : Sum  Inputs=|+-
  Sum2 : Sum  Inputs=|+-
  Sum3 : Sum  Inputs=|++
  Trigonometric Function : Trigonometry
  Trigonometric Function1 : Trigonometry  Operator=cos
  Trigonometric Function2 : Trigonometry
  Trigonometric Function3 : Trigonometry  Operator=cos
  Trigonometric Function4 : Trigonometry
  Trigonometric Function5 : Trigonometry  Operator=cos
  qip : Outport
  wires:
  Selector/1 -> Gain/1
  2/1(inv(q)) -> Quaternion Normalize/1
  orbit/1 -> Selector2/1, Selector1/1, Selector/1
  Selector1/1 -> Gain1/1
  Selector2/1 -> Gain2/1
  Gain/1 -> Trigonometric Function/1, Trigonometric Function1/1
  Gain1/1 -> Trigonometric Function3/1, Trigonometric Function2/1
  Gain2/1 -> Trigonometric Function4/1, Trigonometric Function5/1
  Trigonometric Function1/1 -> Gain3/1, Product2/1, Product5/1, Product7/1
  Gain3/1 -> Product/1
  Trigonometric Function2/1 -> Product/2, Product1/2, Product2/2, Product3/2
  Trigonometric Function5/1 -> Product/3, Product3/3, Product4/3, Product7/3
  Product/1 -> Sum/1
  Trigonometric Function/1 -> Product1/1, Product3/1, Gain4/1
  Trigonometric Function4/1 -> Product1/3, Product2/3, Product5/3, Product6/3
  Product1/1 -> Sum/2
  Product2/1 -> Sum1/1
  Product3/1 -> Sum1/2
  Gain4/1 -> Product4/1, Product6/1
  Trigonometric Function3/1 -> Product4/2, Product5/2, Product6/2, Product7/2
  Product4/1 -> Sum2/1
  Product5/1 -> Sum2/2
  Product6/1 -> Sum3/1
  Product7/1 -> Sum3/2
  Mux/1 -> 2/1(q)
  Quaternion Normalize/1 -> qip/1
  Sum/1 -> Mux/2
  Sum1/1 -> Mux/3
  Sum2/1 -> Mux/4
  Sum3/1 -> Mux/1

== system AA1111/Satellite Software/DataAcquisition/Star sensor measure/2 ==
  Constant : Constant
  Mux : Mux  Inputs=2
  Quaternion Normalize : sharedutil/Quaternion Normalize  aMode=aMode
      settings: SourceProductName=Aerospace Blockset  SourceProductBaseCode=AE
  Random Number1 : RandomNumber  Mean=[0;0;0]  Variance=(Noise_StB*pi/180/3600/3/2).^2  Seed=[2;5;8]  SampleTime=T_ctrl
  q_StBNoise : Outport
  wires:
  Constant/1 -> Mux/1
  Random Number1/1 -> Mux/2
  Quaternion Normalize/1 -> q_StBNoise/1
  Mux/1 -> Quaternion Normalize/1

== system AA1111/Satellite Software/DataAcquisition/Star sensor measure/3 ==
  Constant : Constant
  Demux : Demux
  Mux : Mux  Inputs=2
  Quaternion Normalize : sharedutil/Quaternion Normalize  aMode=aMode
      settings: SourceProductName=Aerospace Blockset  SourceProductBaseCode=AE
  Random Number1 : RandomNumber  Mean=[0;0;0]  Variance=(Noise_StA*pi/180/3600/3/2).^2  Seed=[13;14;15]  SampleTime=T_ctrl
  VoltA1 : Scope  NumInputPorts=4
  q_StANoise : Outport
  wires:
  Mux/1 -> Quaternion Normalize/1, Demux/1
  Quaternion Normalize/1 -> q_StANoise/1
  Random Number1/1 -> Mux/2
  Constant/1 -> Mux/1
  Demux/2 -> VoltA1/2
  Demux/3 -> VoltA1/3
  Demux/4 -> VoltA1/4
  Demux/1 -> VoltA1/1

== system AA1111/Satellite Software/DataAcquisition/Star sensor measure/Q_StA_FixErr ==
  Constant : Constant
  Constant1 : Constant  Value=FixErr_StA/3600/180*pi/2
  Demux : Demux  Outputs=3
  Mux : Mux
  Quaternion Normalize : sharedutil/Quaternion Normalize  aMode=aMode
      settings: SourceProductName=Aerospace Blockset  SourceProductBaseCode=AE
  Q_StA_FixErr : Outport
  wires:
  Mux/1 -> Quaternion Normalize/1
  Quaternion Normalize/1 -> Q_StA_FixErr/1
  Constant1/1 -> Demux/1
  Constant/1 -> Mux/1
  Demux/1 -> Mux/2
  Demux/2 -> Mux/3
  Demux/3 -> Mux/4

== system AA1111/Satellite Software/DataAcquisition/Star sensor measure/Q_StA_FixErr1 ==
  Constant : Constant
  Constant1 : Constant  Value=FixErr_StB/3600/180*pi/2
  Demux : Demux  Outputs=3
  Mux : Mux
  Quaternion Normalize : sharedutil/Quaternion Normalize  aMode=aMode
      settings: SourceProductName=Aerospace Blockset  SourceProductBaseCode=AE
  Q_StB_FixErr : Outport
  wires:
  Demux/3 -> Mux/4
  Demux/2 -> Mux/3
  Demux/1 -> Mux/2
  Constant/1 -> Mux/1
  Constant1/1 -> Demux/1
  Quaternion Normalize/1 -> Q_StB_FixErr/1
  Mux/1 -> Quaternion Normalize/1

== system AA1111/Others/Attitude Kinematics Equations & Attitude Dynamics Equations/Kinetics/EulerIntegral/If Action Subsystem ==
  In1 : Inport
  Action Port : ActionPort  ActionType=then
  EulerDot : MATLABFcn  Priority=1  MATLABFcn=EulerDot  OutputDimensions=3
  Out1 : Outport
  wires:
  In1/1 -> EulerDot/1
  EulerDot/1 -> Out1/1

== system AA1111/Others/Attitude Kinematics Equations & Attitude Dynamics Equations/Kinetics/EulerIntegral/If Action Subsystem1 ==
  In1 : Inport
  Action Port : ActionPort  ActionType=else
  Out1 : Outport
  wires:
  In1/1 -> Out1/1

== system AA1111/Others/Attitude Kinematics Equations & Attitude Dynamics Equations/Kinetics/EulerIntegral1/If Action Subsystem ==
  In1 : Inport
  Action Port : ActionPort  ActionType=then
  EulerDot : MATLABFcn  Priority=1  MATLABFcn=EulerDot  OutputDimensions=3
  Out1 : Outport
  wires:
  EulerDot/1 -> Out1/1
  In1/1 -> EulerDot/1

== system AA1111/Others/Attitude Kinematics Equations & Attitude Dynamics Equations/Kinetics/EulerIntegral1/If Action Subsystem1 ==
  In1 : Inport
  Action Port : ActionPort  ActionType=else
  Out1 : Outport
  wires:
  In1/1 -> Out1/1

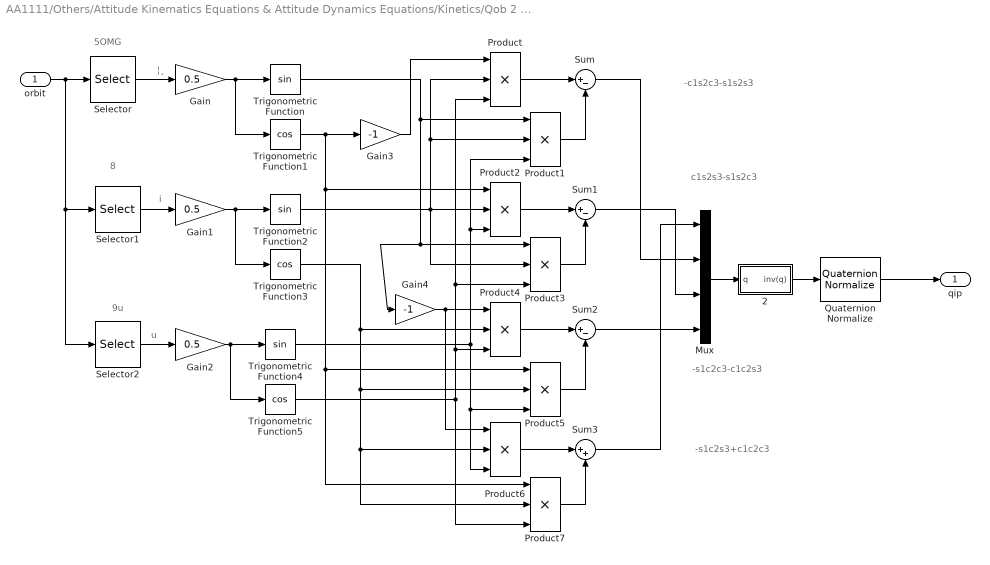
== system AA1111/Others/Attitude Kinematics Equations & Attitude Dynamics Equations/Kinetics/Qob 2 Qib/qip ==
  note: ¦¸
  note: i
  note: u
  note: 5OMG
  note: 8
  note: 9u
  note: -c1s2c3-s1s2s3
  note: c1s2s3-s1s2c3
  note: -s1c2c3-c1c2s3
  note: -s1c2s3+c1c2c3
  orbit : Inport
  2 : Subsystem
      mask Display: disp(' ')
  Gain : Gain  Gain=0.5
  Gain1 : Gain  Gain=0.5
  Gain2 : Gain  Gain=0.5
  Gain3 : Gain  Gain=-1
  Gain4 : Gain  Gain=-1
  Mux : Mux
  Product{,1..7} (8 alike) : Product  Inputs=3  RndMeth=Zero
  Quaternion Normalize : sharedutil/Quaternion Normalize  aMode=aMode
      settings: SourceProductName=Aerospace Blockset  SourceProductBaseCode=AE
  Selector : Selector  InputPortWidth=10  IndexOptions=Index vector (dialog)  Indices=[5]  OutputSizes=1
  Selector1 : Selector  InputPortWidth=10  IndexOptions=Index vector (dialog)  Indices=[8]  OutputSizes=1
  Selector2 : Selector  InputPortWidth=10  IndexOptions=Index vector (dialog)  Indices=[9]  OutputSizes=1
  Sum : Sum  Inputs=|+-
  Sum1 : Sum  Inputs=|+-
  Sum2 : Sum  Inputs=|+-
  Sum3 : Sum  Inputs=|++
  Trigonometric Function : Trigonometry
  Trigonometric Function1 : Trigonometry  Operator=cos
  Trigonometric Function2 : Trigonometry
  Trigonometric Function3 : Trigonometry  Operator=cos
  Trigonometric Function4 : Trigonometry
  Trigonometric Function5 : Trigonometry  Operator=cos
  qip : Outport
  wires:
  Sum3/1 -> Mux/1
  Sum2/1 -> Mux/4
  Sum1/1 -> Mux/3
  Sum/1 -> Mux/2
  Quaternion Normalize/1 -> qip/1
  Mux/1 -> 2/1(q)
  Product7/1 -> Sum3/2
  Product6/1 -> Sum3/1
  Product5/1 -> Sum2/2
  Product4/1 -> Sum2/1
  Trigonometric Function3/1 -> Product7/2, Product6/2, Product5/2, Product4/2
  Gain4/1 -> Product6/1, Product4/1
  Product3/1 -> Sum1/2
  Product2/1 -> Sum1/1
  Product1/1 -> Sum/2
  Trigonometric Function4/1 -> Product6/3, Product5/3, Product2/3, Product1/3
  Trigonometric Function/1 -> Gain4/1, Product3/1, Product1/1
  Product/1 -> Sum/1
  Trigonometric Function5/1 -> Product7/3, Product4/3, Product3/3, Product/3
  Trigonometric Function2/1 -> Product3/2, Product2/2, Product1/2, Product/2
  Gain3/1 -> Product/1
  Trigonometric Function1/1 -> Product7/1, Product5/1, Product2/1, Gain3/1
  Gain2/1 -> Trigonometric Function5/1, Trigonometric Function4/1
  Gain1/1 -> Trigonometric Function2/1, Trigonometric Function3/1
  Gain/1 -> Trigonometric Function1/1, Trigonometric Function/1
  Selector2/1 -> Gain2/1
  Selector1/1 -> Gain1/1
  orbit/1 -> Selector/1, Selector1/1, Selector2/1
  2/1(inv(q)) -> Quaternion Normalize/1
  Selector/1 -> Gain/1

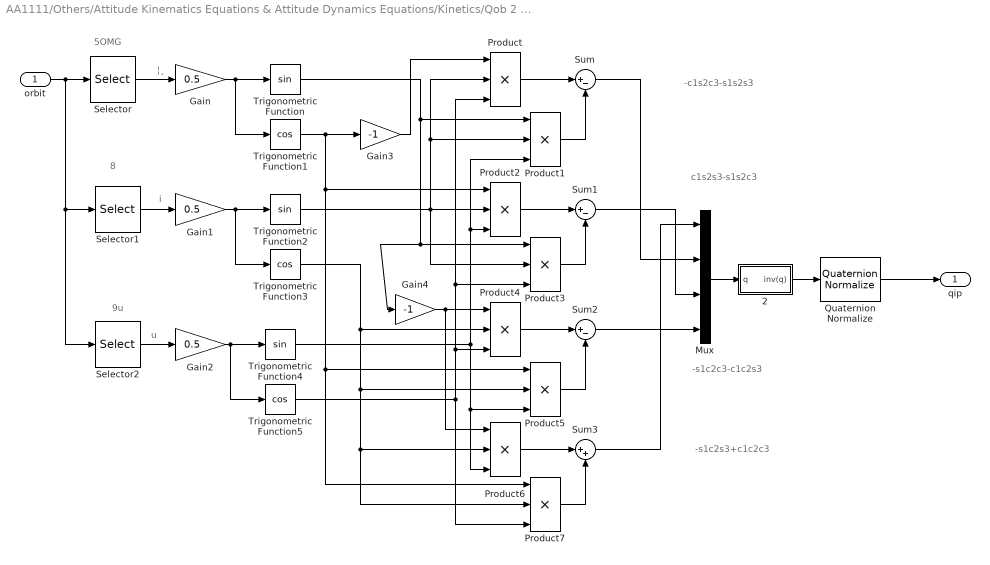
== system AA1111/Others/Attitude Kinematics Equations & Attitude Dynamics Equations/Kinetics/Qob 2 Qib1/qip ==
  note: -s1c2s3+c1c2c3
  note: -s1c2c3-c1c2s3
  note: c1s2s3-s1s2c3
  note: -c1s2c3-s1s2s3
  note: 9u
  note: 8
  note: 5OMG
  note: u
  note: i
  note: ¦¸
  orbit : Inport
  2 : Subsystem
      mask Display: disp(' ')
  Gain : Gain  Gain=0.5
  Gain1 : Gain  Gain=0.5
  Gain2 : Gain  Gain=0.5
  Gain3 : Gain  Gain=-1
  Gain4 : Gain  Gain=-1
  Mux : Mux
  Product{,1..7} (8 alike) : Product  Inputs=3  RndMeth=Zero
  Quaternion Normalize : sharedutil/Quaternion Normalize  aMode=aMode
      settings: SourceProductName=Aerospace Blockset  SourceProductBaseCode=AE
  Selector : Selector  InputPortWidth=10  IndexOptions=Index vector (dialog)  Indices=[5]  OutputSizes=1
  Selector1 : Selector  InputPortWidth=10  IndexOptions=Index vector (dialog)  Indices=[8]  OutputSizes=1
  Selector2 : Selector  InputPortWidth=10  IndexOptions=Index vector (dialog)  Indices=[9]  OutputSizes=1
  Sum : Sum  Inputs=|+-
  Sum1 : Sum  Inputs=|+-
  Sum2 : Sum  Inputs=|+-
  Sum3 : Sum  Inputs=|++
  Trigonometric Function : Trigonometry
  Trigonometric Function1 : Trigonometry  Operator=cos
  Trigonometric Function2 : Trigonometry
  Trigonometric Function3 : Trigonometry  Operator=cos
  Trigonometric Function4 : Trigonometry
  Trigonometric Function5 : Trigonometry  Operator=cos
  qip : Outport
  wires:
  Selector/1 -> Gain/1
  2/1(inv(q)) -> Quaternion Normalize/1
  orbit/1 -> Selector2/1, Selector1/1, Selector/1
  Selector1/1 -> Gain1/1
  Selector2/1 -> Gain2/1
  Gain/1 -> Trigonometric Function/1, Trigonometric Function1/1
  Gain1/1 -> Trigonometric Function3/1, Trigonometric Function2/1
  Gain2/1 -> Trigonometric Function4/1, Trigonometric Function5/1
  Trigonometric Function1/1 -> Gain3/1, Product2/1, Product5/1, Product7/1
  Gain3/1 -> Product/1
  Trigonometric Function2/1 -> Product/2, Product1/2, Product2/2, Product3/2
  Trigonometric Function5/1 -> Product/3, Product3/3, Product4/3, Product7/3
  Product/1 -> Sum/1
  Trigonometric Function/1 -> Product1/1, Product3/1, Gain4/1
  Trigonometric Function4/1 -> Product1/3, Product2/3, Product5/3, Product6/3
  Product1/1 -> Sum/2
  Product2/1 -> Sum1/1
  Product3/1 -> Sum1/2
  Gain4/1 -> Product4/1, Product6/1
  Trigonometric Function3/1 -> Product4/2, Product5/2, Product6/2, Product7/2
  Product4/1 -> Sum2/1
  Product5/1 -> Sum2/2
  Product6/1 -> Sum3/1
  Product7/1 -> Sum3/2
  Mux/1 -> 2/1(q)
  Quaternion Normalize/1 -> qip/1
  Sum/1 -> Mux/2
  Sum1/1 -> Mux/3
  Sum2/1 -> Mux/4
  Sum3/1 -> Mux/1

== system AA1111/Others/Disturbing torque/Compute geomagnetism1/Subsystem/Subsystem1 ==
  note: -2pi~2pi
  note: tan(u)/cos(i)???
  note: ³à¾­
  note: u
  note: Inertia Long.
  note: Geographical Long.
  note: i
  note: OMG
  GAST : Inport
  OrbitElement : Inport  Port=2
  Lat. : Inport  Port=3
  -pi~pi : Subsystem
  -pi~pi1 : Subsystem
  Demux : Demux  Outputs=2
  Fcn1 : Fcn  Expr=cos(u[1])*sin(u[2])/cos(u[3])
  Fcn11 : Fcn  Expr=u(9)
  Fcn2 : Fcn  Expr=rem(u,2*pi)
  Fcn3 : Fcn  Expr=cos(u[2])/cos(u[3])
  Fcn4 : Fcn  Expr=rem(u,2*pi)
  Fcn5 : Fcn  Expr=u(8)
  Fcn9 : Fcn  Expr=u(5)
  If : If  NumInputs=2  IfExpression=u1~=0
  If Action Subsystem1 : Subsystem  TreatAsAtomicUnit=on
  If Action Subsystem2 : Subsystem  TreatAsAtomicUnit=on
  Merge : Merge
  Mux1 : Mux  Inputs=3
  Mux2 : Mux  Inputs=2
  Sum2 : Sum  SaturateOnIntegerOverflow=on
  Sum3 : Sum  Inputs=+-  SaturateOnIntegerOverflow=on
  G_Long. : Outport
  I_Long : Outport  Port=2
  wires:
  Fcn4/1 -> -pi~pi1/1(In1)
  -pi~pi1/1(Out1) -> I_Long/1
  GAST/1 -> Sum3/2
  -pi~pi/1(Out1) -> G_Long./1
  OrbitElement/1 -> Fcn11/1, Fcn5/1, Fcn9/1
  Fcn11/1 -> Mux1/2
  Lat./1 -> Mux1/3
  Mux1/1 -> Fcn1/1, Fcn3/1
  If/1 -> If Action Subsystem2/Action
  Fcn3/1 -> Mux2/1
  Fcn1/1 -> Mux2/2
  Mux2/1 -> Demux/1, If Action Subsystem2/1(In), If Action Subsystem1/1(In)
  Demux/1 -> If/1
  Demux/2 -> If/2
  If Action Subsystem2/1(Out) -> Merge/1
  If/2 -> If Action Subsystem1/Action
  If Action Subsystem1/1(Out) -> Merge/2
  Merge/1 -> Sum2/2
  Sum2/1 -> Fcn4/1, Sum3/1
  Sum3/1 -> Fcn2/1
  Fcn2/1 -> -pi~pi/1(In1)
  Fcn5/1 -> Mux1/1
  Fcn9/1 -> Sum2/1

== system AA1111/Others/Disturbing torque/Compute geomagnetism1/Transfer Matrix/Aop1 ==
  In1 : Inport
  Constant : Constant
  Constant1 : Constant  Value=0
  Gain1 : Gain  Gain=-1
  Mux2 : Mux  Inputs=9
  Reshape : Reshape  OutputDimensionality=Customize  OutputDimensions=[3,3]
  Trigonometric Function : Trigonometry
  Trigonometric Function1 : Trigonometry  Operator=cos
  Out1 : Outport
  wires:
  Trigonometric Function/1 -> Gain1/1, Mux2/2
  Trigonometric Function1/1 -> Mux2/5, Mux2/1
  In1/1 -> Trigonometric Function/1, Trigonometric Function1/1
  Constant1/1 -> Mux2/3, Mux2/6, Mux2/7, Mux2/8
  Constant/1 -> Mux2/9
  Mux2/1 -> Reshape/1
  Reshape/1 -> Out1/1
  Gain1/1 -> Mux2/4

== system AA1111/Others/Disturbing torque/Compute geomagnetism1/Transfer Matrix/If Action Subsystem ==
  In1 : Inport
  Action Port : ActionPort  ActionType=then
  Out1 : Outport
  wires:
  In1/1 -> Out1/1

== system AA1111/Others/Disturbing torque/Compute geomagnetism1/Transfer Matrix/If Action Subsystem1 ==
  In1 : Inport
  Action Port : ActionPort  ActionType=else
  Constant : Constant  Value=pi
  Sum : Sum  Inputs=|-+
  Out1 : Outport
  wires:
  Sum/1 -> Out1/1
  In1/1 -> Sum/1
  Constant/1 -> Sum/2

== system AA1111/Others/Disturbing torque/Compute geomagnetism1/Transfer Matrix/O-NEG ==
  In1 : Inport
  Constant : Constant
  Constant1 : Constant  Value=0
  Gain1 : Gain  Gain=-1
  Mux2 : Mux  Inputs=9
  Reshape : Reshape  OutputDimensionality=Customize  OutputDimensions=[3,3]
  cos3 : Fcn  Expr=sin(u(1))*cos(u(2))/sqrt(1-(sin(u(1)))^2*(sin(u(2)))^2)
  sin : Fcn  Expr=sqrt(1-u(1)^2)
  Out1 : Outport
  wires:
  Gain1/1 -> Mux2/4
  Reshape/1 -> Out1/1
  Mux2/1 -> Reshape/1
  Constant/1 -> Mux2/9
  Constant1/1 -> Mux2/8, Mux2/7, Mux2/6, Mux2/3
  sin/1 -> Mux2/2, Gain1/1
  In1/1 -> cos3/1
  cos3/1 -> Mux2/1, Mux2/5, sin/1

== system AA1111/Others/Oribit motion model/Compute osculating elements/ /If Action Subsystem ==
  note: In+2pi, due to OMG's Range=[0 2*pi],
      | and atan2's Range=[-pi pi]
  In1 : Inport
  Action Port : ActionPort  ActionType=then
  Constant : Constant  Value=2*pi
  Sum : Sum  Inputs=|++  SaturateOnIntegerOverflow=on
  Out1 : Outport
  wires:
  In1/1 -> Sum/1
  Sum/1 -> Out1/1
  Constant/1 -> Sum/2

== system AA1111/Others/Oribit motion model/Compute osculating elements/ /If Action Subsystem1 ==
  In1 : Inport
  Action Port : ActionPort  ActionType=else
  Out1 : Outport
  wires:
  In1/1 -> Out1/1

== system AA1111/Others/Oribit motion model/Compute osculating elements/     /If Action Subsystem2 ==
  In1 : Inport
  Action Port : ActionPort  ActionType=then
  Out1 : Outport
  wires:
  In1/1 -> Out1/1

== system AA1111/Others/Oribit motion model/Compute osculating elements/     /If Action Subsystem3 ==
  In1 : Inport
  Action Port : ActionPort  ActionType=else
  Constant : Constant  Value=2*pi
  Sum : Sum  Inputs=|+-  SaturateOnIntegerOverflow=on
  Out1 : Outport
  wires:
  Sum/1 -> Out1/1
  In1/1 -> Sum/2
  Constant/1 -> Sum/1

== system AA1111/Others/Oribit motion model/Compute osculating elements/     1/If Action Subsystem1 ==
  u : Inport
  T : Inport  Port=2
  Action Port : ActionPort  ActionType=else
  Product : Product  Inputs=3  RndMeth=Zero
  Sum : Sum  Inputs=|+-  SaturateOnIntegerOverflow=on
  uz1 : Constant  Value=pi  VectorParams1D=off
  uz2 : Constant  Value=1/(2*pi)  VectorParams1D=off
  Out1 : Outport
  wires:
  Product/1 -> Out1/1
  uz2/1 -> Product/2
  Sum/1 -> Product/1
  uz1/1 -> Sum/2
  u/1 -> Sum/1
  T/1 -> Product/3
